simulink model "q_2xamd1_stII_q8_usb_DoS"  (R2020b)
settings: Solver=ode4  StartTime=0.0  StopTime=Tend  FixedStep=0.0005  RelTol=1e-3  EnableMultiTasking=on
PostLoadFcn:
  | qc_set_target_type(getConfigSet(bdroot, 'QUARC Default Target Configuration'));
values from neighbouring files (symbols this model uses):
  G = place( A', C', OP )'    [d_2xamd1.m]
  K_AMD_AMP = 1    [Main.m]    (also in Main_setup_stII_2xamd1.m)
  K_AMP = 10    [config_STII.m]
  K_EC = Pr * N_pp / ( 4 * 1024 )    (= 2.27485440932e-05)    [config_2xamd1.m]
  K_ENC = Pb / 8192    [d_STII_sensors.m]
  kd = 2*zeta*Kf*wn    [d_STII_pd.m]
  Kp = ( wn_c^2 * Gc_DEN(1) - Gc_DEN(3) ) / Gc_NUM(1)    [d_2xamd1.m]    (also in d_amd_pv.m)
  kp = wn^2 * Kf    [d_STII_pd.m]
  Kv = ( 2 * zeta_c * wn_c * Gc_DEN(1) - Gc_DEN(2) ) / Gc_NUM(1)    [d_2xamd1.m]    (also in d_amd_pv.m)
  P_MAX = 3.0 * K_IN2M    [config_STII.m]
  SWEEP_MAX = 10e-3    (= 0.01)    [d_shake_table_II.m]
  VMAX_AMP = 13    [config_2xamd1.m]    (also in config_STII.m = 44.1)
  XC_LIM_ENABLE = 1    [Main.m]    (also in Main_setup_stII_2xamd1.m)
  XC_MAX = 0.08    [Main.m]    (also in Main_setup_stII_2xamd1.m)
  XC_MIN = - XC_MAX    (= -0.08)    [Main.m]    (also in Main_setup_stII_2xamd1.m)
undefined symbols (not defined in the file or in its folder): A, B, C, D, HIL, K_G2MS, K_MS2G, Kamd, qc_get_step_size, VMAX_AMP_AMD
libraries: quarc_library x29, simulink x9
settings Model: SimulationMode=external  ExtModeTrigDuration=10000  Creator=MLevis  LastModifiedBy=aleja
settings SolverCC: PositivePriorityOrder=on
settings DataIOCC: LimitDataPoints=on  SaveFormat=Array  SignalLoggingSaveFormat=ModelDataLogs  ReturnWorkspaceOutputs=off
settings OptimizationCC: InitFltsAndDblsToZero=on  LifeSpan=inf
settings DebuggingCC: SaveWithParameterizedLinksMsg=none  UnderspecifiedInitializationDetection=Classic  MergeDetectMultiDrivingBlocksExec=none  SolverPrmCheckMsg=warning  MultiTaskDSMMsg=warning  MultiTaskCondExecSysMsg=none  FcnCallInpInsideContextMsg=warning  StateNameClashWarn=warning  SFUnexpectedBacktrackingDiag=warning  SFNoUnconditionalDefaultTransitionDiag=warning  ArithmeticOperatorsInVariantConditions=warning
settings HardwareCC: ProdBitPerPointer=32  ProdBitPerSizeT=32  ProdBitPerPtrDiffT=32  ProdLargestAtomicFloat=None  ProdIntDivRoundTo=Undefined  ProdEndianess=Unspecified  ProdWordSize=32  ProdHWDeviceType=32-bit Generic
settings ModelReferenceCC: PropagateSignalLabelsOutOfModel=off
settings SFSimCC: SimUseLocalCustomCode=off  CustomCodeUndefinedFunction=UseInterfaceOnly
settings RTWCC: Description=QUARC Win64 Target  SystemTargetFile=quarc_win64.tlc  TemplateMakefile=quarc_default_tmf  RTWUseLocalCustomCode=off
settings CodeAppCC: StateflowObjectComments=on
settings STFCustomTargetCC: TargetPreCompLibLocation=C:\PROGRA~3\QUARC\lib\2019b\win64\release  CombineOutputUpdateFcns=on  CPPClassGenCompliant=off  GRTInterface=off
settings GRTTargetCC: TargetPreCompLibLocation=C:\PROGRA~3\QUARC\lib\2019b\win64\release  TargetLangStandard=C89/C90 (ANSI)  ParMdlRefBuildCompliant=off  CompOptLevelCompliant=off  MatFileLogging=off  CPPClassGenCompliant=off  UseToolchainInfoCompliant=off  ExtMode=on  ExtModeMexFile=quarc_comm
settings ConfigComp: CovMetricSettings=dw  CovSaveCumulativeToWorkspaceVar=on  CovSaveSingleToWorkspaceVar=on  CovExternalEMLEnable=off  CovSFcnEnable=off

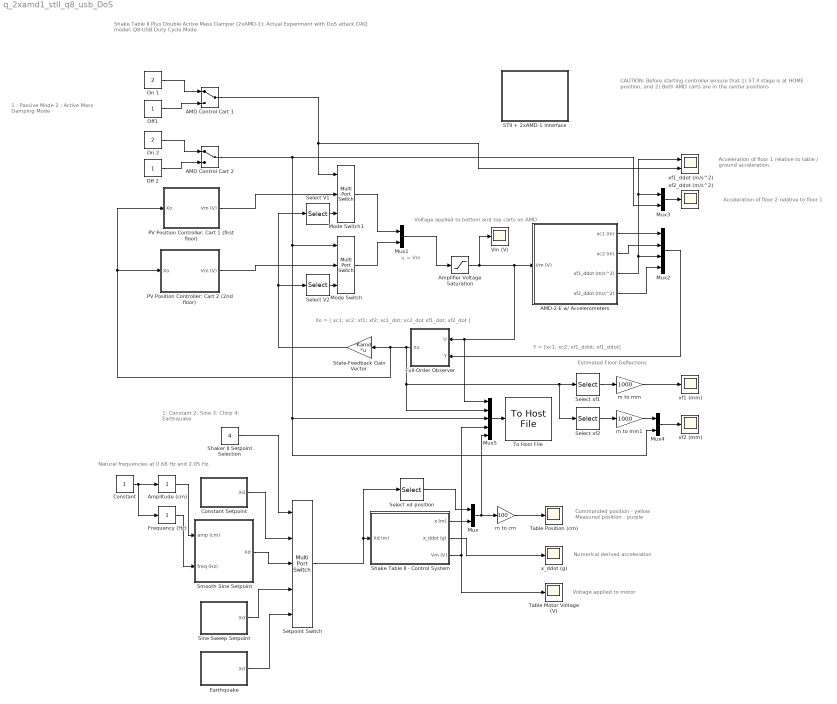
== system q_2xamd1_stII_q8_usb_DoS ==
  note: Natural frequencies at 0.68 Hz and 2.05 Hz.
  note: Shake Table II Plus Double Active Mass Damper (2xAMD-1): Actual Experiment with DoS attack
      | DAQ model: Q8-USB
      | Duty Cycle Mode
  note: CAUTION:
      | Before starting controller ensure that
      | 1) ST II stage is at HOME position, and
      | 2) Both AMD carts are in the center positions
  note: 1: Constant
      | 2: Sine
      | 3: Chirp
      | 4: Earthquake
  note: Commanded position - yellow
      | Measured position - purple
  note: Voltage applied to motor
  note: Numerical derived acceleration
  note: u = Vm
  note: Xo = [ xc1; xc2; xf1; xf2; xc1_dot; xc2_dot xf1_dot; xf2_dot ]
  note: Y = [xc1; xc2; xf1_ddot; xf1_ddot]
  note: 1 : Passive Mode
      | 2 : Active Mass Damping Mode
  note: Acceleration of floor 1 relative to table /
      | ground acceleration.
  note: Acceleration of floor 2 relative to floor 1
  note: Voltage applied to bottom and top carts on AMD
  note: Estimated Floor Deflections
  AMD Control Cart 1 : ManualSwitch
  AMD Control Cart 2 : ManualSwitch
  "AMD-2-E w/ Accelerometers " : Subsystem
  Amplifier Voltage Saturation : Saturate  UpperLimit=VMAX_AMP_AMD  LowerLimit=- VMAX_AMP_AMD
  Amplitude (cm) : simulink/Math Operations/Slider Gain  gain=1  low=0  high=5
  Constant : Constant
  Constant Setpoint : Subsystem
  Earthquake : Subsystem
  Frequency (Hz) : simulink/Math Operations/Slider Gain  gain=1  low=0  high=3.5
  Full-Order Observer : Subsystem
  Mode Switch : MultiPortSwitch  Inputs=2  SaturateOnIntegerOverflow=on  InputSameDT=on
  Mode Switch1 : MultiPortSwitch  Inputs=2  SaturateOnIntegerOverflow=on  InputSameDT=on
  Mux{,1,3..4} (4 alike) : Mux  Inputs=2
  Mux2 : Mux
  Mux5 : Mux  Inputs=5
  Off 2 : Constant
  Off1 : Constant
  On 1 : Constant  Value=2
  On 2 : Constant  Value=2
  PV Position Controller: Cart 1 (first floor) : Subsystem
  PV Position Controller: Cart 2 (2nd floor) : Subsystem
  STII + 2xAMD-1 Interface : Subsystem
  Select V1 : Selector  InputPortWidth=2  IndexOptions=Index vector (dialog)  Indices=[1]  OutputSizes=1
  Select V2 : Selector  InputPortWidth=2  IndexOptions=Index vector (dialog)  Indices=[2]  OutputSizes=1
  Select xd position : Selector  InputPortWidth=2  IndexOptions=Index vector (dialog)  Indices=1  OutputSizes=1
  Select xf1 : Selector  InputPortWidth=8  IndexOptions=Index vector (dialog)  Indices=3  OutputSizes=1
  Select xf2 : Selector  InputPortWidth=8  IndexOptions=Index vector (dialog)  Indices=4  OutputSizes=1
  Setpoint Switch : MultiPortSwitch  Inputs=4  SaturateOnIntegerOverflow=on  InputSameDT=on
  Shake Table II - Control System : Subsystem
  Shaker II Setpoint Selection : Constant  Value=4
  Sine Sweep Setpoint : Subsystem
  Smooth Sine Setpoint : Subsystem
  State-Feedback Gain Vector : Gain  Gain=-Kamd  Multiplication=Matrix(K*u)  SaturateOnIntegerOverflow=on  OutDataTypeStr=Inherit: Same as input  ParamDataTypeStr=Inherit: Same as input
  Table Motor Voltage (V) : Scope
  Table Position (cm) : Scope
  To Host File : quarc_library/Sinks/To Host/To Host File  file_name=sample_data_stII_2xamd01.mat  variable_name=data  decimation=1  sample_time=-1  file_format=MAT-file v.4  options=No header or footer  append=off  final_file_name=sample_data_stII_2xamd01.mat  bitrate=2000000
  Vm (V) : Scope
  m to cm : Gain  Gain=100
  m to mm : Gain  Gain=1000
  m to mm1 : Gain  Gain=1000
  x_ddot (g) : Scope
  xf1 (mm) : Scope
  xf1_ddot (m/s^2) : Scope  NumInputPorts=2
  xf2 (mm) : Scope
  xf2_ddot (m/s^2) : Scope
  wires:
  Setpoint Switch/1 -> Select xd position/1, Shake Table II - Control System/1(Xd (m))
  Shaker II Setpoint Selection/1 -> Setpoint Switch/1
  Constant Setpoint/1(Xd) -> Setpoint Switch/2
  Sine Sweep Setpoint/1(Xd) -> Setpoint Switch/4
  Constant/1 -> Amplitude (cm)/1, Frequency (Hz)/1
  Amplitude (cm)/1 -> Smooth Sine Setpoint/1(amp (cm))
  Frequency (Hz)/1 -> Smooth Sine Setpoint/2(freq (Hz))
  Smooth Sine Setpoint/1(Xd) -> Setpoint Switch/3
  Shake Table II - Control System/1(x (m)) -> Mux/2
  Mux/1 -> Mux5/5, m to cm/1
  m to cm/1 -> Table Position (cm)/1
  Select xd position/1 -> Mux/1
  Shake Table II - Control System/3(Vm (V)) -> Table Motor Voltage (V)/1, Mux5/4
  Shake Table II - Control System/2(x_ddot (g)) -> x_ddot (g)/1
  Mux2/1 -> Full-Order Observer/2(Y)
  "AMD-2-E w/ Accelerometers "/1(xc1 (m)) -> Mux2/1
  "AMD-2-E w/ Accelerometers "/2(xc2 (m)) -> Mux2/2
  "AMD-2-E w/ Accelerometers "/3(xf1_ddot (m/s^2)) -> Mux3/1, xf1_ddot (m/s^2)/1, Mux2/3
  "AMD-2-E w/ Accelerometers "/4(xf2_ddot (m/s^2)) -> Mux2/4
  On 2/1 -> AMD Control Cart 2/1
  Off 2/1 -> AMD Control Cart 2/2
  AMD Control Cart 2/1 -> Mux5/3, Mux4/2, Mode Switch/1, Mux3/2
  Select xf1/1 -> m to mm/1
  Full-Order Observer/1(Xo) -> State-Feedback Gain Vector/1, PV Position Controller: Cart 2 (2nd floor)/1(Xo), PV Position Controller: Cart 1 (first floor)/1(Xo), Mux5/2, Select xf2/1, Select xf1/1
  Select xf2/1 -> m to mm1/1
  m to mm/1 -> xf1 (mm)/1
  Amplifier Voltage Saturation/1 -> Vm (V)/1, Mux5/1, Full-Order Observer/1(U), "AMD-2-E w/ Accelerometers "/1(Vm (V))
  Mux3/1 -> xf2_ddot (m/s^2)/1
  m to mm1/1 -> Mux4/1
  Mux4/1 -> xf2 (mm)/1
  Mux5/1 -> To Host File/1
  Off1/1 -> AMD Control Cart 1/2
  On 1/1 -> AMD Control Cart 1/1
  Mode Switch1/1 -> Mux1/1
  Mode Switch/1 -> Mux1/2
  Mux1/1 -> Amplifier Voltage Saturation/1
  PV Position Controller: Cart 1 (first floor)/1(Vm (V)) -> Mode Switch1/2
  PV Position Controller: Cart 2 (2nd floor)/1(Vm (V)) -> Mode Switch/2
  AMD Control Cart 1/1 -> xf1_ddot (m/s^2)/2, Mode Switch1/1
  Earthquake/1(Xd) -> Setpoint Switch/5
  State-Feedback Gain Vector/1 -> Select V1/1, Select V2/1
  Select V2/1 -> Mode Switch/3
  Select V1/1 -> Mode Switch1/3

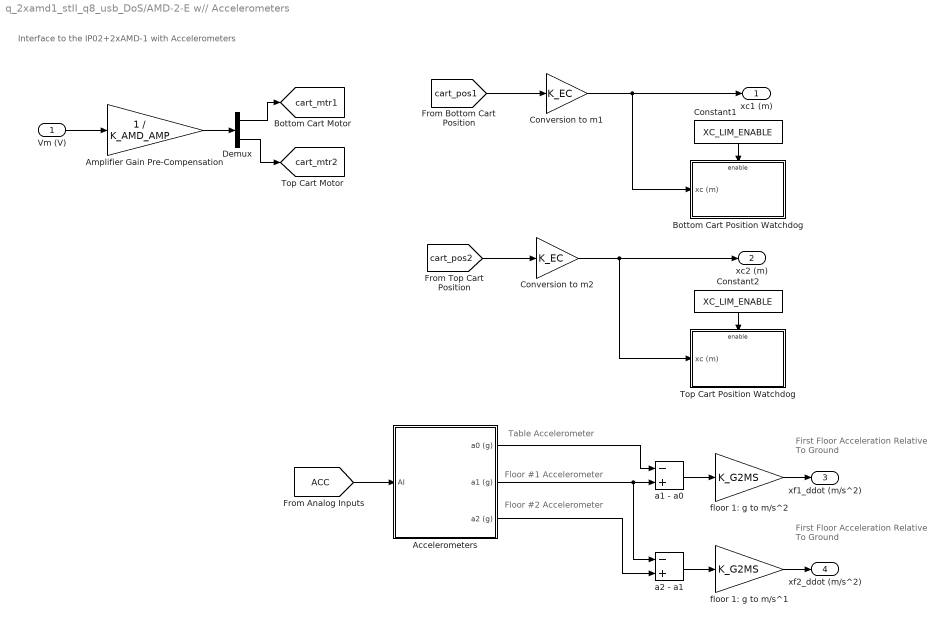
== system q_2xamd1_stII_q8_usb_DoS/AMD-2-E w// Accelerometers  ==
  note: First Floor Acceleration
      | Relative To Ground
  note: First Floor Acceleration
      | Relative To Ground
  note: Floor #2 Accelerometer
  note: Floor #1 Accelerometer
  note: Table Accelerometer
  note: Interface to the IP02+2xAMD-1 with Accelerometers
  Vm (V) : Inport
  Accelerometers : Subsystem  Description=Accelerometer Module
  Amplifier Gain Pre-Compensation : Gain  Gain=1 / K_AMD_AMP  SaturateOnIntegerOverflow=on  OutDataTypeStr=Inherit: Same as input  ParamDataTypeStr=Inherit: Same as input
  Bottom Cart Position Watchdog : Subsystem  TreatAsAtomicUnit=on
  Constant1 : Constant  Value=XC_LIM_ENABLE
  Constant2 : Constant  Value=XC_LIM_ENABLE
  Conversion to m1 : Gain  Gain=K_EC  SaturateOnIntegerOverflow=on  OutDataTypeStr=Inherit: Same as input  ParamDataTypeStr=Inherit: Same as input
  Conversion to m2 : Gain  Gain=K_EC  SaturateOnIntegerOverflow=on  OutDataTypeStr=Inherit: Same as input  ParamDataTypeStr=Inherit: Same as input
  Demux : Demux  Outputs=2
  Top Cart Position Watchdog : Subsystem  TreatAsAtomicUnit=on
  a1 - a0 : Sum  Inputs=-+
  a2 - a1 : Sum  Inputs=-+
  floor 1: g to m/s^1 : Gain  Gain=K_G2MS  SaturateOnIntegerOverflow=on  OutDataTypeStr=Inherit: Same as input  ParamDataTypeStr=Inherit: Same as input
  floor 1: g to m/s^2 : Gain  Gain=K_G2MS  SaturateOnIntegerOverflow=on  OutDataTypeStr=Inherit: Same as input  ParamDataTypeStr=Inherit: Same as input
  xc1 (m) : Outport  VectorParamsAs1DForOutWhenUnconnected=off
  xc2 (m) : Outport  Port=2  VectorParamsAs1DForOutWhenUnconnected=off
  xf1_ddot (m/s^2) : Outport  Port=3  InitialOutput=0  VectorParamsAs1DForOutWhenUnconnected=off
  xf2_ddot (m/s^2) : Outport  Port=4  InitialOutput=0  VectorParamsAs1DForOutWhenUnconnected=off
  tag scope: cart_mtr1=global, cart_mtr2=global
  wires:
  [ACC] -> Accelerometers/1(AI)
  floor 1: g to m/s^1/1 -> xf2_ddot (m/s^2)/1
  a2 - a1/1 -> floor 1: g to m/s^1/1
  Accelerometers/3(a2 (g)) -> a2 - a1/2
  Accelerometers/2(a1 (g)) -> a2 - a1/1, a1 - a0/2
  Accelerometers/1(a0 (g)) -> a1 - a0/1
  floor 1: g to m/s^2/1 -> xf1_ddot (m/s^2)/1
  a1 - a0/1 -> floor 1: g to m/s^2/1
  Vm (V)/1 -> Amplifier Gain Pre-Compensation/1
  Demux/1 -> [cart_mtr1]
  Demux/2 -> [cart_mtr2]
  Constant2/1 -> Top Cart Position Watchdog/Enable
  Conversion to m2/1 -> xc2 (m)/1, Top Cart Position Watchdog/1(xc (m))
  Conversion to m1/1 -> xc1 (m)/1, Bottom Cart Position Watchdog/1(xc (m))
  [cart_pos1] -> Conversion to m1/1
  [cart_pos2] -> Conversion to m2/1
  Constant1/1 -> Bottom Cart Position Watchdog/Enable
  Amplifier Gain Pre-Compensation/1 -> Demux/1

== system q_2xamd1_stII_q8_usb_DoS/Constant Setpoint ==
  Mux2 : Mux  Inputs=2
  Position Setpoint (m) : Constant  Value=0
  Velocity Setpoint (m/s) : Constant  Value=0
  Xd : Outport  VectorParamsAs1DForOutWhenUnconnected=off
  wires:
  Position Setpoint (m)/1 -> Mux2/1
  Velocity Setpoint (m/s)/1 -> Mux2/2
  Mux2/1 -> Xd/1

== system q_2xamd1_stII_q8_usb_DoS/Earthquake ==
  note: Position Setpoint
  Continuous Sigmoid : quarc_library/Sources/Sigmoids/Continuous Sigmoid  params_source=Internal (dialog parameters)  max_velocity=VEL_MAX  max_acceleration=ACC_MAX  initial_position=0  initial_velocity=0  hold_off=0.1  input_sample_time=-1  output_sample_time=qc_get_step_size
      settings: SourceProductName=QUARC Targets
  Mux2 : Mux  Inputs=2
  Position Limit : Saturate  UpperLimit=P_MAX  LowerLimit=-P_MAX
  Repeating Sequence Interpolated : simulink/Sources/Repeating Sequence Interpolated  OutValues=xd  TimeValues=Tc  LookUpMeth=Interpolation-Use End Values  tsamp=qc_get_step_size  OutMin=[]  OutMax=[]  OutDataTypeStr=float('double')  OutputDataTypeScalingMode=Specify via dialog  OutDataType=float('double')  OutScaling=2^-10
  Terminator : Terminator
  Terminator1 : Terminator
  Velocity Setpoint Weight : simulink/Math Operations/Slider Gain  gain=1  low=0  high=1
  Xd : Outport
  wires:
  Continuous Sigmoid/1 -> Mux2/1
  Continuous Sigmoid/4 -> Terminator1/1
  Continuous Sigmoid/3 -> Terminator/1
  Repeating Sequence Interpolated/1 -> Position Limit/1
  Mux2/1 -> Xd/1
  Velocity Setpoint Weight/1 -> Mux2/2
  Position Limit/1 -> Continuous Sigmoid/1
  Continuous Sigmoid/2 -> Velocity Setpoint Weight/1

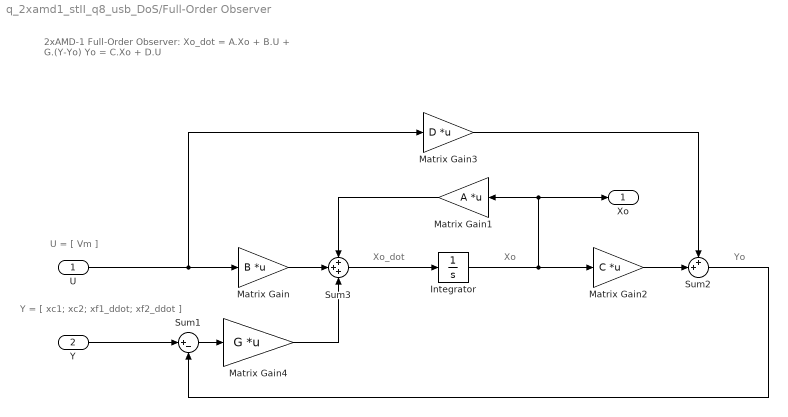
== system q_2xamd1_stII_q8_usb_DoS/Full-Order Observer ==
  note: U = [ Vm ]
  note: 2xAMD-1 Full-Order Observer:
      | Xo_dot = A.Xo + B.U + G.(Y-Yo)
      | Yo = C.Xo + D.U
  note: Y = [ xc1; xc2; xf1_ddot; xf2_ddot ]
  note: Xo
  note: Xo_dot
  note: Yo
  U : Inport
  Y : Inport  Port=2
  Integrator : Integrator
  Matrix Gain : Gain  Gain=B  Multiplication=Matrix(K*u)  SaturateOnIntegerOverflow=on  OutDataTypeStr=Inherit: Same as input  ParamDataTypeStr=Inherit: Same as input
  Matrix Gain1 : Gain  Gain=A  Multiplication=Matrix(K*u)  SaturateOnIntegerOverflow=on  OutDataTypeStr=Inherit: Same as input  ParamDataTypeStr=Inherit: Same as input
  Matrix Gain2 : Gain  Gain=C  Multiplication=Matrix(K*u)  SaturateOnIntegerOverflow=on  OutDataTypeStr=Inherit: Same as input  ParamDataTypeStr=Inherit: Same as input
  Matrix Gain3 : Gain  Gain=D  Multiplication=Matrix(K*u)  SaturateOnIntegerOverflow=on  OutDataTypeStr=Inherit: Same as input  ParamDataTypeStr=Inherit: Same as input
  Matrix Gain4 : Gain  Gain=G  Multiplication=Matrix(K*u)  SaturateOnIntegerOverflow=on  OutDataTypeStr=Inherit: Same as input  ParamDataTypeStr=Inherit: Same as input
  Sum1 : Sum  Inputs=|+-  InputSameDT=on  SaturateOnIntegerOverflow=on  OutDataTypeStr=Inherit: Same as first input
  Sum2 : Sum  Inputs=++|  InputSameDT=on  SaturateOnIntegerOverflow=on  OutDataTypeStr=Inherit: Same as first input
  Sum3 : Sum  Inputs=+++  InputSameDT=on  SaturateOnIntegerOverflow=on  OutDataTypeStr=Inherit: Same as first input
  Xo : Outport  VectorParamsAs1DForOutWhenUnconnected=off
  wires:
  Y/1 -> Sum1/1
  U/1 -> Matrix Gain/1, Matrix Gain3/1
  Matrix Gain/1 -> Sum3/2
  Sum3/1 -> Integrator/1
  Integrator/1 -> Xo/1, Matrix Gain1/1, Matrix Gain2/1
  Matrix Gain2/1 -> Sum2/2
  Matrix Gain3/1 -> Sum2/1
  Matrix Gain1/1 -> Sum3/1
  Sum1/1 -> Matrix Gain4/1
  Matrix Gain4/1 -> Sum3/3
  Sum2/1 -> Sum1/2

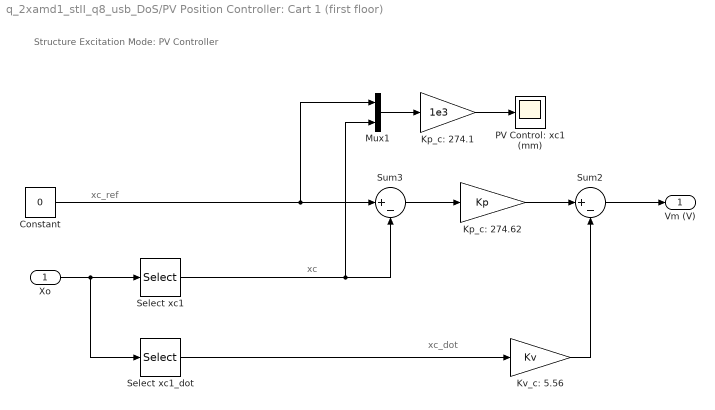
== system q_2xamd1_stII_q8_usb_DoS/PV Position Controller: Cart 1 (first floor) ==
  note: Structure Excitation Mode:
      | PV Controller
  note: xc_ref
  note: xc_dot
  note: xc
  Xo : Inport
  Constant : Constant  Value=0
  Kp_c: 274.1 : Gain  Gain=1e3  SaturateOnIntegerOverflow=on  OutDataTypeStr=Inherit: Same as input  ParamDataTypeStr=Inherit: Same as input
  Kp_c: 274.62 : Gain  Gain=Kp  SaturateOnIntegerOverflow=on  OutDataTypeStr=Inherit: Same as input  ParamDataTypeStr=Inherit: Same as input
  Kv_c: 5.56 : Gain  Gain=Kv  SaturateOnIntegerOverflow=on  OutDataTypeStr=Inherit: Same as input  ParamDataTypeStr=Inherit: Same as input
  Mux1 : Mux  Inputs=2
  PV Control: xc1 (mm) : Scope
  Select xc1 : Selector  InputPortWidth=8  IndexOptions=Index vector (dialog)  Indices=[1]  OutputSizes=1
  Select xc1_dot : Selector  InputPortWidth=8  IndexOptions=Index vector (dialog)  Indices=[5]  OutputSizes=1
  Sum2 : Sum  Inputs=|+-  InputSameDT=on  SaturateOnIntegerOverflow=on  OutDataTypeStr=Inherit: Same as first input
  Sum3 : Sum  Inputs=|+-  InputSameDT=on  SaturateOnIntegerOverflow=on  OutDataTypeStr=Inherit: Same as first input
  Vm (V) : Outport  VectorParamsAs1DForOutWhenUnconnected=off
  wires:
  Kp_c: 274.62/1 -> Sum2/1
  Kv_c: 5.56/1 -> Sum2/2
  Select xc1_dot/1 -> Kv_c: 5.56/1
  Sum3/1 -> Kp_c: 274.62/1
  Constant/1 -> Mux1/1, Sum3/1
  Sum2/1 -> Vm (V)/1
  Mux1/1 -> Kp_c: 274.1/1
  Select xc1/1 -> Sum3/2, Mux1/2
  Kp_c: 274.1/1 -> PV Control: xc1 (mm)/1
  Xo/1 -> Select xc1/1, Select xc1_dot/1

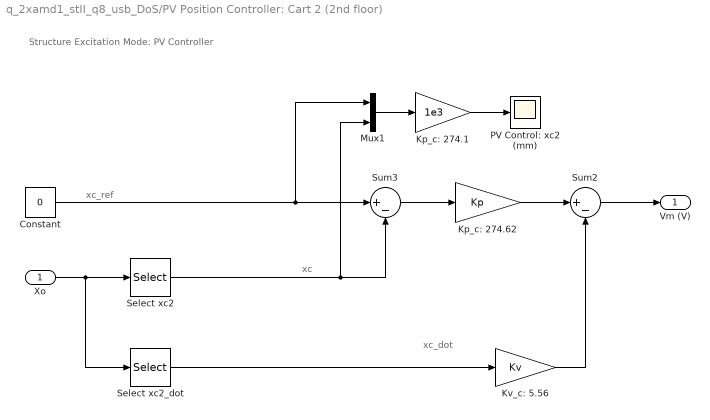
== system q_2xamd1_stII_q8_usb_DoS/PV Position Controller: Cart 2 (2nd floor) ==
  note: xc
  note: xc_dot
  note: xc_ref
  note: Structure Excitation Mode:
      | PV Controller
  Xo : Inport
  Constant : Constant  Value=0
  Kp_c: 274.1 : Gain  Gain=1e3  SaturateOnIntegerOverflow=on  OutDataTypeStr=Inherit: Same as input  ParamDataTypeStr=Inherit: Same as input
  Kp_c: 274.62 : Gain  Gain=Kp  SaturateOnIntegerOverflow=on  OutDataTypeStr=Inherit: Same as input  ParamDataTypeStr=Inherit: Same as input
  Kv_c: 5.56 : Gain  Gain=Kv  SaturateOnIntegerOverflow=on  OutDataTypeStr=Inherit: Same as input  ParamDataTypeStr=Inherit: Same as input
  Mux1 : Mux  Inputs=2
  PV Control: xc2 (mm) : Scope
  "Select xc2 " : Selector  InputPortWidth=8  IndexOptions=Index vector (dialog)  Indices=[2]  OutputSizes=1
  Select xc2_dot : Selector  InputPortWidth=8  IndexOptions=Index vector (dialog)  Indices=[6]  OutputSizes=1
  Sum2 : Sum  Inputs=|+-  InputSameDT=on  SaturateOnIntegerOverflow=on  OutDataTypeStr=Inherit: Same as first input
  Sum3 : Sum  Inputs=|+-  InputSameDT=on  SaturateOnIntegerOverflow=on  OutDataTypeStr=Inherit: Same as first input
  Vm (V) : Outport  VectorParamsAs1DForOutWhenUnconnected=off
  wires:
  Xo/1 -> "Select xc2 "/1, Select xc2_dot/1
  Kp_c: 274.1/1 -> PV Control: xc2 (mm)/1
  "Select xc2 "/1 -> Mux1/2, Sum3/2
  Mux1/1 -> Kp_c: 274.1/1
  Sum2/1 -> Vm (V)/1
  Constant/1 -> Sum3/1, Mux1/1
  Sum3/1 -> Kp_c: 274.62/1
  Select xc2_dot/1 -> Kv_c: 5.56/1
  Kv_c: 5.56/1 -> Sum2/2
  Kp_c: 274.62/1 -> Sum2/1

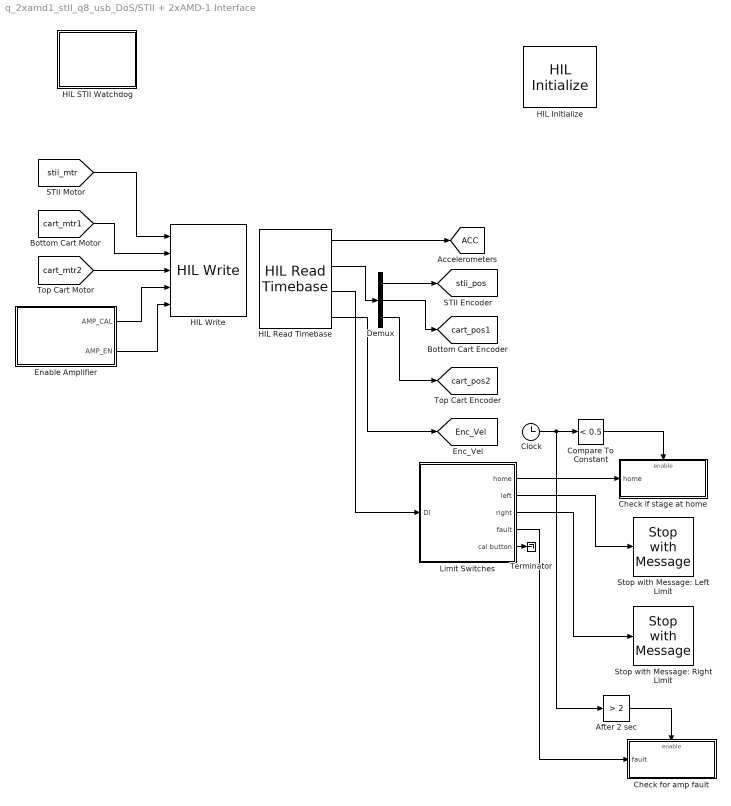
== system q_2xamd1_stII_q8_usb_DoS/STII + 2xAMD-1 Interface ==
  After 2 sec : simulink/Logic and Bit Operations/Compare To Constant  relop=>  const=2  OutDataTypeStr=uint8  ZeroCross=off
  Check for amp fault : Subsystem  TreatAsAtomicUnit=on
  Check if stage at home : Subsystem  TreatAsAtomicUnit=on
  Clock : Clock
  Compare To Constant : simulink/Logic and Bit Operations/Compare To Constant  relop=<  const=0.5  OutDataTypeStr=uint8  ZeroCross=off
  Demux : Demux  Outputs=3
  Enable Amplifier : Subsystem
  HIL Initialize : quarc_library/Data Acquisition/Generic/Configuration/HIL Initialize  object_name=HIL-1  board_type=q8_usb  board_number=0  board_options=update_rate=fast;ext_int_polarity=0;convert_polarity=1;watchdog_polarity=0;ext_int_watchdog=0;use_convert=0;pwm_immediate=0;decimation=1  exclusive=off  active=on  hardware_clocks=[0:2]  clock_modes=[]  initial_clock_frequencies=[]  set_clock_params_at_start=off  set_clock_params_at_switch_in=off  set_clock_frequencies_at_start=off  set_clock_frequencies_at_switch_in=off  analog_input_channels=[0:7]  analog_input_configurations=[]  analog_input_maximums=10  analog_input_minimums=-10  set_analog_input_params_at_start=on  set_analog_input_params_at_switch_in=off  analog_output_channels=[0:7]  analog_output_maximums=10  analog_output_minimums=-10  initial_analog_outputs=[0]  final_analog_outputs=[0]  watchdog_analog_outputs=0  set_analog_output_params_at_start=on  set_analog_output_params_at_switch_in=off  set_analog_outputs_at_start=on  set_analog_outputs_at_switch_in=off  set_analog_outputs_at_terminate=on  set_analog_outputs_at_switch_out=off  set_analog_outputs_on_watchdog=on  digital_input_channels=[0:4]  digital_output_channels=[0:7]  digital_output_configuration=[]  initial_digital_outputs=[0]  final_digital_outputs=[0]  watchdog_digital_outputs=[0]  set_digital_output_params_at_start=off  set_digital_output_params_at_switch_in=off  set_digital_outputs_at_start=on  set_digital_outputs_at_switch_in=off  set_digital_outputs_at_terminate=on  set_digital_outputs_at_switch_out=off  set_digital_outputs_on_watchdog=on  encoder_channels=[0:7]  quadrature=[4]  encoder_filter_frequency=[]  initial_encoder_counts=[0]  set_encoder_params_at_start=on  set_encoder_params_at_switch_in=off  set_encoder_counts_at_start=on  set_encoder_counts_at_switch_in=off  pwm_channels=[0:7]  pwm_modes=0  pwm_frequency=99.532799999999995e6/4095  pwm_configuration=[0]  pwm_alignment=[0]  pwm_polarity=[1]  pwm_leading_deadband=[0]  pwm_trailing_deadband=[0]  initial_pwm_outputs=[0]  final_pwm_outputs=[0]  watchdog_pwm_outputs=[0]  set_pwm_params_at_start=on  set_pwm_params_at_switch_in=off  set_pwm_outputs_at_start=on  set_pwm_outputs_at_switch_in=off  set_pwm_outputs_at_terminate=on  set_pwm_outputs_at_switch_out=off  set_pwm_outputs_on_watchdog=off  other_output_channels=[]  initial_other_outputs=[]  final_other_outputs=[]  watchdog_other_outputs=[]  set_other_outputs_at_start=off  set_other_outputs_at_switch_in=off  set_other_outputs_at_terminate=off  set_other_outputs_at_switch_out=off  set_other_outputs_on_watchdog=off
  HIL Read Timebase : quarc_library/Data Acquisition/Generic/Timebases/HIL Read Timebase  object_name=HIL-1  clock=0  analog_channels=[0:2]  encoder_channels=[0:2]  digital_channels=[0:4]  other_channels=[14000]  samples_in_buffer=max(ceil(1/qc_get_step_size), 1)  active=on  vector_output=on  data_type_mode=Inherit via back propagation  encoder_data_type=double  digital_data_type=boolean
  HIL STII Watchdog : Subsystem
  HIL Write : quarc_library/Data Acquisition/Generic/Immediate I//O/HIL Write  object_name=HIL-1  analog_channels=[0:2]  pwm_channels=[]  digital_channels=[0:1]  other_channels=[]  sample_time=-1  active=off  vector_input=off
  Limit Switches : Subsystem
  Stop with Message: Left Limit : quarc_library/Sinks/Error Handling/Stop with Message  message_type=Fixed error message  message_icon=Error  message=Left limit switch has been triggered!
  Stop with Message: Right Limit : quarc_library/Sinks/Error Handling/Stop with Message  message_type=Fixed error message  message_icon=Error  message=Right limit switch has been triggered!
  Terminator : Terminator
  tag scope: ACC=global, Enc_Vel=global, cart_pos1=global, cart_pos2=global, stii_pos=global
  wires:
  Demux/1 -> [stii_pos]
  HIL Read Timebase/1 -> [ACC]
  Demux/2 -> [cart_pos1]
  [cart_mtr1] -> HIL Write/2
  [cart_mtr2] -> HIL Write/3
  Demux/3 -> [cart_pos2]
  Enable Amplifier/2("AMP_EN ") -> HIL Write/5
  HIL Read Timebase/2 -> Demux/1
  Limit Switches/1(home) -> Check if stage at home/1(home)
  Clock/1 -> After 2 sec/1, Compare To Constant/1
  Limit Switches/3(right) -> Stop with Message: Right Limit/1
  Limit Switches/2(left) -> Stop with Message: Left Limit/1
  Compare To Constant/1 -> Check if stage at home/Enable
  Limit Switches/5(cal button) -> Terminator/1
  After 2 sec/1 -> Check for amp fault/Enable
  Limit Switches/4(fault) -> Check for amp fault/1(fault)
  HIL Read Timebase/3 -> Limit Switches/1(DI)
  [stii_mtr] -> HIL Write/1
  Enable Amplifier/1(AMP_CAL) -> HIL Write/4
  HIL Read Timebase/4 -> [Enc_Vel]

== system q_2xamd1_stII_q8_usb_DoS/Shake Table II - Control System ==
  Xd (m) : Inport
  Position Controller : Subsystem
  "Shake Table II " : Subsystem
  x (m) : Outport  InitialOutput=0  VectorParamsAs1DForOutWhenUnconnected=off
  x_ddot (g) : Outport  Port=2  VectorParamsAs1DForOutWhenUnconnected=off
  Vm (V) : Outport  Port=3  InitialOutput=0  VectorParamsAs1DForOutWhenUnconnected=off
  wires:
  "Shake Table II "/2(x_dot (m/s)) -> Position Controller/2(x_dot (m/s))
  Position Controller/1(u (A)) -> "Shake Table II "/1(u (V))
  Xd (m)/1 -> Position Controller/3(Xd)
  "Shake Table II "/4(Vm (V)) -> Vm (V)/1
  "Shake Table II "/1(x (m)) -> x (m)/1, Position Controller/1(x (m))
  "Shake Table II "/3(x_ddot (g)) -> x_ddot (g)/1

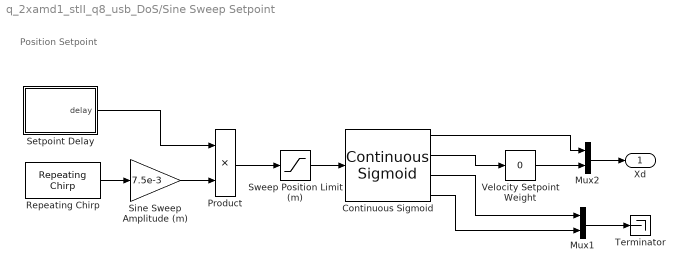
== system q_2xamd1_stII_q8_usb_DoS/Sine Sweep Setpoint ==
  note: Position Setpoint
  Continuous Sigmoid : quarc_library/Sources/Sigmoids/Continuous Sigmoid  params_source=Internal (dialog parameters)  max_velocity=VEL_MAX  max_acceleration=ACC_MAX  initial_position=0  initial_velocity=0  hold_off=0.1  input_sample_time=-1  output_sample_time=qc_get_step_size
      settings: SourceProductName=QUARC Targets
  Mux1 : Mux  Inputs=2
  Mux2 : Mux  Inputs=2
  Product : Product  RndMeth=Zero
  Repeating Chirp : quarc_library/Sources/Signals/Repeating Chirp  Description=Special Chirsp . starts and stops with zero...  A=1  f1=0.1  T=19  f2=3.5  D=1
      settings: SourceProductName=QUARC Targets
  Setpoint Delay : Subsystem
  Sine Sweep Amplitude (m) : Gain  Gain=7.5e-3
  Sweep Position Limit (m) : Saturate  UpperLimit=SWEEP_MAX  LowerLimit=-SWEEP_MAX
  Terminator : Terminator
  Velocity Setpoint Weight : simulink/Math Operations/Slider Gain  gain=0  low=0  high=1
  Xd : Outport  VectorParamsAs1DForOutWhenUnconnected=off
  wires:
  Mux1/1 -> Terminator/1
  Mux2/1 -> Xd/1
  Velocity Setpoint Weight/1 -> Mux2/2
  Continuous Sigmoid/1 -> Mux2/1
  Sweep Position Limit (m)/1 -> Continuous Sigmoid/1
  Repeating Chirp/1 -> Sine Sweep Amplitude (m)/1
  Setpoint Delay/1(delay) -> Product/1
  Sine Sweep Amplitude (m)/1 -> Product/2
  Product/1 -> Sweep Position Limit (m)/1
  Continuous Sigmoid/2 -> Velocity Setpoint Weight/1
  Continuous Sigmoid/3 -> Mux1/1
  Continuous Sigmoid/4 -> Mux1/2

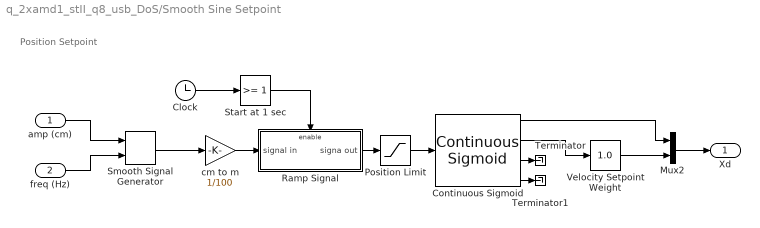
== system q_2xamd1_stII_q8_usb_DoS/Smooth Sine Setpoint ==
  note: Position Setpoint
  amp (cm) : Inport
  freq (Hz) : Inport  Port=2
  Clock : Clock
  Continuous Sigmoid : quarc_library/Sources/Sigmoids/Continuous Sigmoid  params_source=Internal (dialog parameters)  max_velocity=VEL_MAX  max_acceleration=ACC_MAX  initial_position=0  initial_velocity=0  hold_off=0.1  input_sample_time=-1  output_sample_time=qc_get_step_size
      settings: SourceProductName=QUARC Targets
  Mux2 : Mux  Inputs=2
  Position Limit : Saturate  UpperLimit=P_MAX  LowerLimit=-P_MAX
  Ramp Signal : Subsystem  TreatAsAtomicUnit=on
  Smooth Signal Generator : quarc_library/Sources/Signals/Smooth Signal Generator  signal_type=Sine  source=External (input ports)  amplitude=1  frequency=1  initial_phase=0  sample_time=qc_get_step_size  output_cos=off
      settings: SourceProductName=QUARC Targets
  Start at 1 sec : simulink/Logic and Bit Operations/Compare To Constant  relop=>=  const=1  OutDataTypeStr=boolean
  Terminator : Terminator
  Terminator1 : Terminator
  Velocity Setpoint Weight : simulink/Math Operations/Slider Gain  gain=1.0  low=0  high=1
  cm to m : Gain  Gain=1/100
  Xd : Outport  VectorParamsAs1DForOutWhenUnconnected=off
  wires:
  Ramp Signal/1(signa out) -> Position Limit/1
  cm to m/1 -> Ramp Signal/1(signal in)
  Smooth Signal Generator/1 -> cm to m/1
  Position Limit/1 -> Continuous Sigmoid/1
  Continuous Sigmoid/1 -> Mux2/1
  Continuous Sigmoid/2 -> Velocity Setpoint Weight/1
  Velocity Setpoint Weight/1 -> Mux2/2
  Mux2/1 -> Xd/1
  freq (Hz)/1 -> Smooth Signal Generator/2
  amp (cm)/1 -> Smooth Signal Generator/1
  Continuous Sigmoid/3 -> Terminator/1
  Continuous Sigmoid/4 -> Terminator1/1
  Start at 1 sec/1 -> Ramp Signal/Enable
  Clock/1 -> Start at 1 sec/1

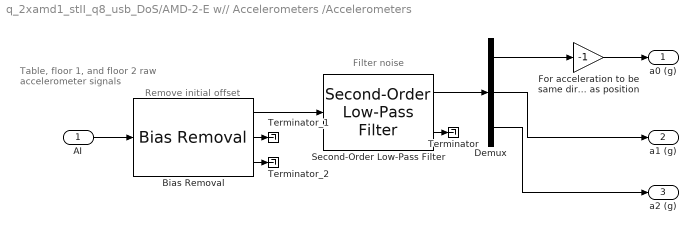
== system q_2xamd1_stII_q8_usb_DoS/AMD-2-E w// Accelerometers /Accelerometers ==
  note: Table, floor 1, and floor 2 raw accelerometer signals
  note: Remove initial offset
  note: Filter noise
  AI : Inport
  Bias Removal : quarc_library/Discrete/Bias Removal  start_time=0  end_time=0.1  switch_id=0  sample_time=qc_get_step_size
      settings: SourceProductName=QUARC Targets
  Demux : Demux  Outputs=3
  For acceleration to be same direction as position : Gain  Gain=-1
  Second-Order Low-Pass Filter : quarc_library/Continuous/Second-Order Low-Pass Filter  params_source=Internal (dialog parameters)  input_width=wa  input_zeta=za  input_init=0
  Terminator : Terminator
  Terminator_1 : Terminator
  Terminator_2 : Terminator
  a0 (g) : Outport  InitialOutput=0  VectorParamsAs1DForOutWhenUnconnected=off
  a1 (g) : Outport  Port=2  InitialOutput=0  VectorParamsAs1DForOutWhenUnconnected=off
  a2 (g) : Outport  Port=3  InitialOutput=0  VectorParamsAs1DForOutWhenUnconnected=off
  wires:
  Second-Order Low-Pass Filter/2 -> Terminator/1
  Demux/3 -> a2 (g)/1
  Demux/2 -> a1 (g)/1
  Demux/1 -> For acceleration to be same direction as position/1
  For acceleration to be same direction as position/1 -> a0 (g)/1
  AI/1 -> Bias Removal/1
  Bias Removal/3 -> Terminator_2/1
  Bias Removal/2 -> Terminator_1/1
  Bias Removal/1 -> Second-Order Low-Pass Filter/1
  Second-Order Low-Pass Filter/1 -> Demux/1

== system q_2xamd1_stII_q8_usb_DoS/AMD-2-E w// Accelerometers /Bottom Cart Position Watchdog ==
  xc (m) : Inport
  Enable : EnablePort
  Check Maximum Allowed Position : RelationalOperator  Operator=<  RndMeth=Nearest  InputSameDT=on
  Check Minimum Allowed Position : RelationalOperator  Operator=<  RndMeth=Nearest  InputSameDT=on
  Stop with Message : quarc_library/Sinks/Error Handling/Stop with Message  message_type=Fixed error message  message_icon=Error  message=Bottom cart: maximum limit reached.
  Stop with Message1 : quarc_library/Sinks/Error Handling/Stop with Message  message_type=Fixed error message  message_icon=Error  message=Bottom cart: minimum limit reached.
  X IN : Constant  Value=XC_MIN
  X MAX : Constant  Value=XC_MAX
  wires:
  Check Maximum Allowed Position/1 -> Stop with Message/1
  xc (m)/1 -> Check Minimum Allowed Position/1, Check Maximum Allowed Position/2
  X IN/1 -> Check Minimum Allowed Position/2
  Check Minimum Allowed Position/1 -> Stop with Message1/1
  X MAX/1 -> Check Maximum Allowed Position/1

== system q_2xamd1_stII_q8_usb_DoS/AMD-2-E w// Accelerometers /Top Cart Position Watchdog ==
  xc (m) : Inport
  Enable : EnablePort
  Check Maximum Allowed Position : RelationalOperator  Operator=<  RndMeth=Nearest  InputSameDT=on
  Check Minimum Allowed Position : RelationalOperator  Operator=<  RndMeth=Nearest  InputSameDT=on
  Stop with Message : quarc_library/Sinks/Error Handling/Stop with Message  message_type=Fixed error message  message_icon=Error  message=Top cart: maximum limit reached.
  Stop with Message1 : quarc_library/Sinks/Error Handling/Stop with Message  message_type=Fixed error message  message_icon=Error  message=Top cart: minimum limit reached.
  X IN : Constant  Value=XC_MIN
  X MAX : Constant  Value=XC_MAX
  wires:
  X MAX/1 -> Check Maximum Allowed Position/1
  Check Minimum Allowed Position/1 -> Stop with Message1/1
  X IN/1 -> Check Minimum Allowed Position/2
  xc (m)/1 -> Check Maximum Allowed Position/2, Check Minimum Allowed Position/1
  Check Maximum Allowed Position/1 -> Stop with Message/1

== system q_2xamd1_stII_q8_usb_DoS/STII + 2xAMD-1 Interface/Check for amp fault ==
  fault : Inport
  Enable : EnablePort
  Stop with Message: Amp Fault : quarc_library/Sinks/Error Handling/Stop with Message  message_type=Fixed error message  message_icon=Error  message=AMPAQ-PWM fault.
  wires:
  fault/1 -> Stop with Message: Amp Fault/1

== system q_2xamd1_stII_q8_usb_DoS/STII + 2xAMD-1 Interface/Check if stage at home ==
  home : Inport
  Enable : EnablePort
  Logical Operator : Logic  Operator=NOT  AllPortsSameDT=off  OutDataTypeStr=boolean
  Stop with Message : quarc_library/Sinks/Error Handling/Stop with Message  message_type=Fixed error message  message_icon=Error  message=Error Table not at home. Calibrate table before starting this controller.
  wires:
  Logical Operator/1 -> Stop with Message/1
  home/1 -> Logical Operator/1

== system q_2xamd1_stII_q8_usb_DoS/STII + 2xAMD-1 Interface/Enable Amplifier ==
  Calibrate Signal = OFF : Constant  Value=0  OutDataTypeStr=boolean
  Enable Signal = ON : Constant  OutDataTypeStr=boolean
  AMP_CAL : Outport  InitialOutput=[0]  VectorParamsAs1DForOutWhenUnconnected=off
  "AMP_EN " : Outport  Port=2  VectorParamsAs1DForOutWhenUnconnected=off
  wires:
  Calibrate Signal = OFF/1 -> AMP_CAL/1
  Enable Signal = ON/1 -> "AMP_EN "/1

== system q_2xamd1_stII_q8_usb_DoS/STII + 2xAMD-1 Interface/HIL STII Watchdog ==
  HIL Watchdog : quarc_library/Data Acquisition/Generic/Watchdog/HIL Watchdog  object_name=HIL-1  timeout=hil_timeout  sample_time=qc_get_step_size  active=off
      settings: AttributesFormatString=(%<object_name>)  SourceProductName=QUARC Targets
  Stop with Error : quarc_library/Sinks/Error Handling/Stop with Error  message_type=Fixed error message  message=Stopped by Watchdog - controller began running too slow.
      settings: AttributesFormatString="\"%<message>\""  SourceProductName=QUARC Targets
  wires:
  HIL Watchdog/1 -> Stop with Error/1

== system q_2xamd1_stII_q8_usb_DoS/STII + 2xAMD-1 Interface/Limit Switches ==
  DI : Inport
  Demux : Demux  Outputs=5
  debouncer: left : quarc_library/Discontinuities/Debouncer  init_state=Off  param_src=Specify via dialog  threshold=dbnc_threshold  rise_time=dbnc_rise_time  fall_time=0
      settings: SourceProductName=QUARC Targets
  debouncer: right : quarc_library/Discontinuities/Debouncer  init_state=Off  param_src=Specify via dialog  threshold=dbnc_threshold  rise_time=dbnc_rise_time  fall_time=0
      settings: SourceProductName=QUARC Targets
  home : Outport  VectorParamsAs1DForOutWhenUnconnected=off
  left : Outport  Port=2  VectorParamsAs1DForOutWhenUnconnected=off
  right : Outport  Port=3  VectorParamsAs1DForOutWhenUnconnected=off
  fault : Outport  Port=4  VectorParamsAs1DForOutWhenUnconnected=off
  cal button : Outport  Port=5  VectorParamsAs1DForOutWhenUnconnected=off
  wires:
  Demux/5 -> cal button/1
  debouncer: right/1 -> right/1
  Demux/3 -> debouncer: right/1
  DI/1 -> Demux/1
  Demux/2 -> home/1
  Demux/4 -> fault/1
  Demux/1 -> debouncer: left/1
  debouncer: left/1 -> left/1

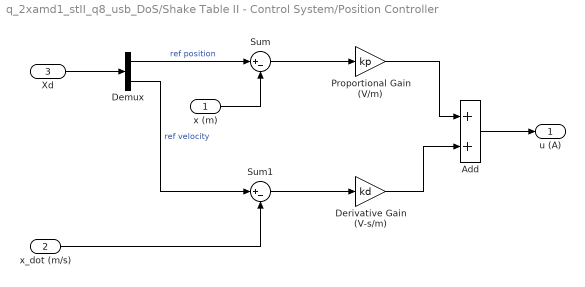
== system q_2xamd1_stII_q8_usb_DoS/Shake Table II - Control System/Position Controller ==
  x (m) : Inport
  x_dot (m/s) : Inport  Port=2
  Xd : Inport  Port=3
  Add : Sum
  Demux : Demux  Outputs=2
  Derivative Gain (V-s/m) : Gain  Gain=kd
  Proportional Gain (V/m) : Gain  Gain=kp
  Sum : Sum  Inputs=|+-
  Sum1 : Sum  Inputs=|+-
  u (A) : Outport  VectorParamsAs1DForOutWhenUnconnected=off
  wires:
  Add/1 -> u (A)/1
  Proportional Gain (V/m)/1 -> Add/1
  Derivative Gain (V-s/m)/1 -> Add/2
  Sum1/1 -> Derivative Gain (V-s/m)/1
  Sum/1 -> Proportional Gain (V/m)/1
  x_dot (m/s)/1 -> Sum1/2
  Demux/2 -> Sum1/1  "ref velocity"
  x (m)/1 -> Sum/2
  Demux/1 -> Sum/1  "ref position"
  Xd/1 -> Demux/1

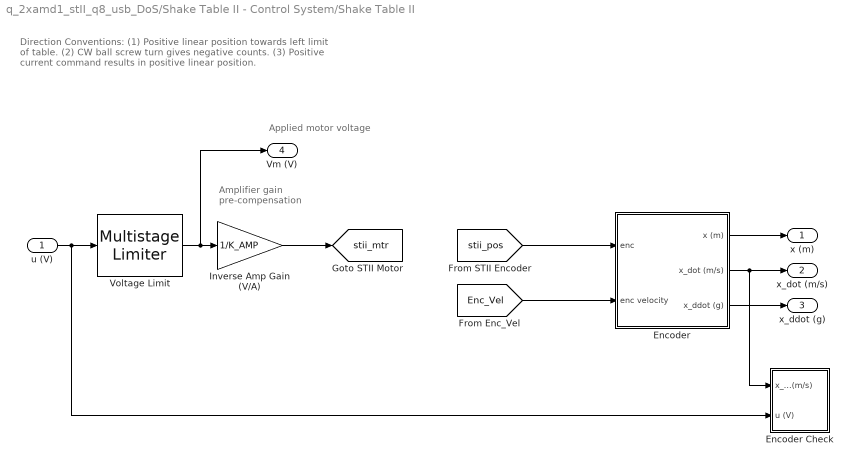
== system q_2xamd1_stII_q8_usb_DoS/Shake Table II - Control System/Shake Table II  ==
  note: Amplifier gain
      | pre-compensation
  note: Direction Conventions:
      | (1) Positive linear position towards left limit of table.
      | (2) CW ball screw turn gives negative counts.
      | (3) Positive current command results in positive linear position.
  note: Applied motor voltage
  u (V) : Inport
  Encoder : Subsystem
  Encoder Check : Subsystem
  Inverse Amp Gain (V/A) : Gain  Gain=1/K_AMP  SaturateOnIntegerOverflow=on  OutDataTypeStr=Inherit: Same as input  ParamDataTypeStr=Inherit: Same as input
  Voltage Limit : quarc_library/Discontinuities/Multistage Limiter  peak_lim=VMAX_AMP  peak_time_lim=2  cont_lim=VMAX_AMP/2  cont_hold_time=1
      settings: SourceProductName=QUARC Targets
  x (m) : Outport  InitialOutput=0  VectorParamsAs1DForOutWhenUnconnected=off
  x_dot (m/s) : Outport  Port=2  InitialOutput=0  VectorParamsAs1DForOutWhenUnconnected=off
  x_ddot (g) : Outport  Port=3  InitialOutput=0  VectorParamsAs1DForOutWhenUnconnected=off
  Vm (V) : Outport  Port=4  InitialOutput=0  VectorParamsAs1DForOutWhenUnconnected=off
  tag scope: stii_mtr=global
  wires:
  Encoder/2(x_dot (m/s)) -> Encoder Check/1(x_dot (m/s)), x_dot (m/s)/1
  Encoder/3(x_ddot (g)) -> x_ddot (g)/1
  Encoder/1(x (m)) -> x (m)/1
  [Enc_Vel] -> Encoder/2(enc velocity)
  [stii_pos] -> Encoder/1(enc)
  Voltage Limit/1 -> Inverse Amp Gain (V/A)/1, Vm (V)/1
  u (V)/1 -> Encoder Check/2(u (V)), Voltage Limit/1
  Inverse Amp Gain (V/A)/1 -> [stii_mtr]

== system q_2xamd1_stII_q8_usb_DoS/Sine Sweep Setpoint/Setpoint Delay ==
  note: UPM not enabled until after 0.7 s.
      | Only generate setpoint after 1.0 s.
  Clock : Clock
  Data Type Conversion : DataTypeConversion
  Discretized Transfer Function : quarc_library/Discrete/Discretized Transfer Function  num=[1]  den=[1 1]  method=tustin  Ts=qc_get_step_size
      settings: SourceProductName=QUARC Targets
  Relational Operator : RelationalOperator  OutDataTypeStr=boolean  RndMeth=Nearest
  UPM Init Time (s) : Constant  Value=1.0
  delay : Outport  VectorParamsAs1DForOutWhenUnconnected=off
  wires:
  Data Type Conversion/1 -> Discretized Transfer Function/1
  Discretized Transfer Function/1 -> delay/1
  Relational Operator/1 -> Data Type Conversion/1
  Clock/1 -> Relational Operator/1
  UPM Init Time (s)/1 -> Relational Operator/2

== system q_2xamd1_stII_q8_usb_DoS/Smooth Sine Setpoint/Ramp Signal ==
  signal in : Inport
  Enable : EnablePort
  Constant : Constant  SampleTime=qc_get_step_size
  Gain : Gain  Gain=2
  Integrator : Integrator
  Product : Product
  Sum : Sum  Inputs=|+-
  signa out : Outport  VectorParamsAs1DForOutWhenUnconnected=off
  wires:
  Integrator/1 -> Sum/2, Product/2
  Sum/1 -> Gain/1
  Constant/1 -> Sum/1
  Gain/1 -> Integrator/1
  Product/1 -> signa out/1
  signal in/1 -> Product/1

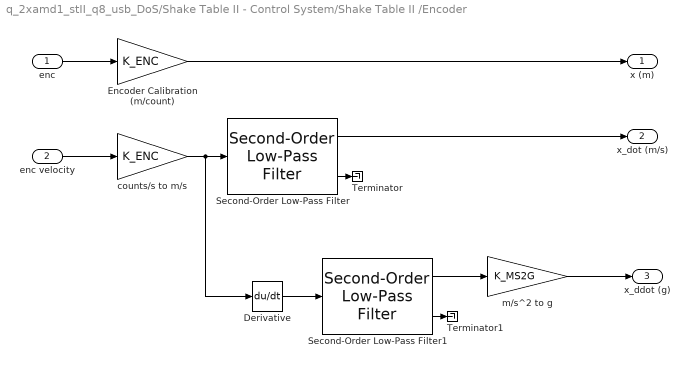
== system q_2xamd1_stII_q8_usb_DoS/Shake Table II - Control System/Shake Table II /Encoder ==
  enc : Inport
  enc velocity : Inport  Port=2
  Derivative : Derivative
  Encoder Calibration (m/count) : Gain  Gain=K_ENC  SaturateOnIntegerOverflow=on  OutDataTypeStr=Inherit: Same as input  ParamDataTypeStr=Inherit: Same as input
  Second-Order Low-Pass Filter : quarc_library/Continuous/Second-Order Low-Pass Filter  params_source=Internal (dialog parameters)  input_width=wd  input_zeta=zd  input_init=0
  Second-Order Low-Pass Filter1 : quarc_library/Continuous/Second-Order Low-Pass Filter  params_source=Internal (dialog parameters)  input_width=wa  input_zeta=za  input_init=0
  Terminator : Terminator
  Terminator1 : Terminator
  counts/s to m/s : Gain  Gain=K_ENC  SaturateOnIntegerOverflow=on  OutDataTypeStr=Inherit: Same as input  ParamDataTypeStr=Inherit: Same as input
  m/s^2 to g : Gain  Gain=K_MS2G
  x (m) : Outport  InitialOutput=0  VectorParamsAs1DForOutWhenUnconnected=off
  x_dot (m/s) : Outport  Port=2  InitialOutput=0  VectorParamsAs1DForOutWhenUnconnected=off
  x_ddot (g) : Outport  Port=3  InitialOutput=0  VectorParamsAs1DForOutWhenUnconnected=off
  wires:
  Second-Order Low-Pass Filter/1 -> x_dot (m/s)/1
  Second-Order Low-Pass Filter1/2 -> Terminator1/1
  Second-Order Low-Pass Filter/2 -> Terminator/1
  Second-Order Low-Pass Filter1/1 -> m/s^2 to g/1
  counts/s to m/s/1 -> Second-Order Low-Pass Filter/1, Derivative/1
  enc velocity/1 -> counts/s to m/s/1
  m/s^2 to g/1 -> x_ddot (g)/1
  Derivative/1 -> Second-Order Low-Pass Filter1/1
  Encoder Calibration (m/count)/1 -> x (m)/1
  enc/1 -> Encoder Calibration (m/count)/1

== system q_2xamd1_stII_q8_usb_DoS/Shake Table II - Control System/Shake Table II /Encoder Check ==
  x_dot (m/s) : Inport
  u (V) : Inport  Port=2
  Abs : Abs
  Abs1 : Abs
  Display : Display
  Encoder not reading : quarc_library/Sinks/Error Handling/Stop with Message  message_type=Fixed error message  message_icon=Error  message=Current applied and not reading position. Check E-Stop and verify encoder is working.
  Rate Transition : RateTransition
  Stall Monitor : quarc_library/Discrete/Stall Monitor  control_threshold=0.7  motion_threshold=0.001  duration_s=.05
      settings: SourceProductName=QUARC Targets
  wires:
  Abs/1 -> Stall Monitor/1
  u (V)/1 -> Abs/1
  Stall Monitor/2 -> Encoder not reading/1
  x_dot (m/s)/1 -> Abs1/1
  Abs1/1 -> Rate Transition/1
  Rate Transition/1 -> Stall Monitor/2
  Stall Monitor/1 -> Display/1
